simulink model "mdl_1_newLogic"  (R2016a)
settings: Solver=FixedStepAuto  StartTime=0.0  StopTime=10.0  RelTol=1e-3
settings Model: Creator=chrysler2  LastModifiedBy=chrysler2
settings GRTTargetCC: GeneratePreprocessorConditionals=Use local settings

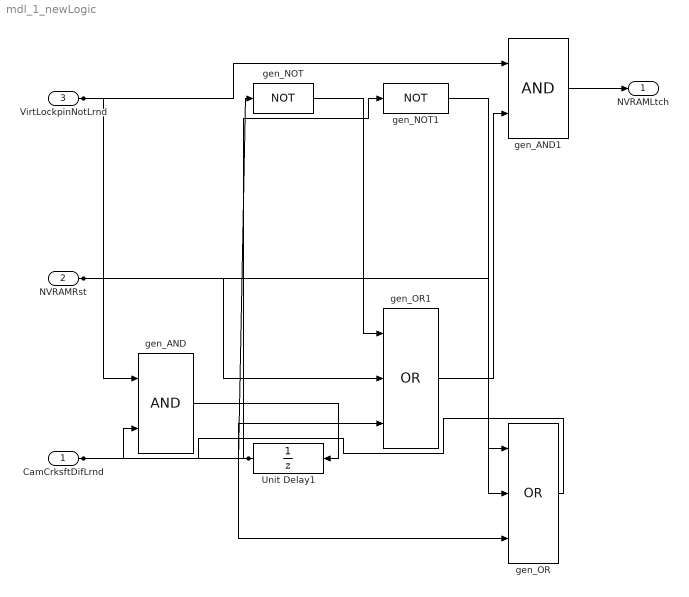
== system mdl_1_newLogic ==
  CamCrksftDifLrnd : Inport
  NVRAMRst : Inport  Port=2
  VirtLockpinNotLrnd : Inport  Port=3
  Unit Delay1 : UnitDelay  SampleTime=-1
  gen_AND : Logic
  gen_AND1 : Logic
  gen_NOT : Logic  Operator=NOT
  gen_NOT1 : Logic  Operator=NOT
  gen_OR : Logic  Operator=OR  Inputs=3
  gen_OR1 : Logic  Operator=OR  Inputs=3
  NVRAMLtch : Outport
  wires:
  CamCrksftDifLrnd/1 -> gen_NOT/1, gen_NOT1/1
  NVRAMRst/1 -> gen_OR/2, gen_OR1/2
  Unit Delay1/1 -> gen_OR/3, gen_OR1/3
  VirtLockpinNotLrnd/1 -> gen_AND/1, gen_AND1/1
  gen_AND/1 -> Unit Delay1/1
  gen_OR/1 -> gen_AND/2
  gen_OR1/1 -> gen_AND1/2
  gen_NOT1/1 -> gen_OR/1
  gen_NOT/1 -> gen_OR1/1
  gen_AND1/1 -> NVRAMLtch/1
